simulink model "Simple_4Quad_payload_02"  (R2018b)
settings: Solver=VariableStepAuto  StartTime=0.0  StopTime=60  RelTol=1e-3
InitFcn:
  | Simple_4Quad_payload_02_const
values from neighbouring files (symbols this model uses):
  d1 = 0.25    [Colab_4Quad_model_01_const.m]    (also in Colab_4Quad_model_02_const.m = 0.5; Simple_4Quad_payload_01_const.m = 1; Simple_4Quad_payload_02_const.m = 1; Simple_4Quad_payload_03_const.m = 1)
  d2 = 0.25    [Colab_4Quad_model_01_const.m]    (also in Colab_4Quad_model_02_const.m = 0.5; Simple_4Quad_payload_01_const.m = 1; Simple_4Quad_payload_02_const.m = 1; Simple_4Quad_payload_03_const.m = 1)
  Des_rel_dist = 2    [Simple_4Quad_payload_01_const.m]    (also in Simple_4Quad_payload_02_const.m = 4; Simple_4Quad_payload_03_const.m = 4; Simple_4Quad_payload_04_const.m; Simple_4Quad_payload_05_const.m)
  g = 9.81    [Colab_4Quad_model_01_const.m]    (also in Colab_4Quad_model_02_const.m; Simple_2Quad_payload_01_const.m; Simple_2Quad_payload_02_const.m; Simple_2Quad_payload_03_const.m)
  Ix = 0.166667    [Colab_4Quad_model_01_const.m]    (also in Colab_4Quad_model_02_const.m = 0.02; Simple_4Quad_payload_01_const.m = 1; Simple_4Quad_payload_02_const.m = 1; Simple_4Quad_payload_03_const.m = 1)
  Iy = 0.166667    [Colab_4Quad_model_01_const.m]    (also in Colab_4Quad_model_02_const.m = 0.02; Simple_4Quad_payload_01_const.m = 1; Simple_4Quad_payload_02_const.m = 1; Simple_4Quad_payload_03_const.m = 1)
  Iz = 0.166667    [Colab_4Quad_model_01_const.m]    (also in Colab_4Quad_model_02_const.m = 0.02; Simple_4Quad_payload_01_const.m = 1; Simple_4Quad_payload_02_const.m = 1; Simple_4Quad_payload_03_const.m = 1)
  ki1_N = 0    [Simple_4Quad_payload_02_const.m]    (also in Simple_4Quad_payload_03_const.m; Simple_4Quad_payload_04_const.m; Simple_4Quad_payload_05_const.m; Simple_4Quad_payload_06_const.m)
  ki1_S = 0    [Simple_4Quad_payload_02_const.m]    (also in Simple_4Quad_payload_03_const.m; Simple_4Quad_payload_04_const.m)
  ki2_N = 0    [Simple_4Quad_payload_02_const.m]    (also in Simple_4Quad_payload_03_const.m; Simple_4Quad_payload_04_const.m; Simple_4Quad_payload_05_const.m; Simple_4Quad_payload_06_const.m = 10)
  ki2_S = 0    [Simple_4Quad_payload_02_const.m]    (also in Simple_4Quad_payload_03_const.m; Simple_4Quad_payload_04_const.m)
  kp1_N = 10    [Simple_4Quad_payload_02_const.m]    (also in Simple_4Quad_payload_03_const.m; Simple_4Quad_payload_04_const.m; Simple_4Quad_payload_05_const.m = 1; Simple_4Quad_payload_06_const.m = 1)
  kp1_S = 10    [Simple_4Quad_payload_02_const.m]    (also in Simple_4Quad_payload_03_const.m; Simple_4Quad_payload_04_const.m)
  kp2_N = 100    [Simple_4Quad_payload_02_const.m]    (also in Simple_4Quad_payload_03_const.m; Simple_4Quad_payload_04_const.m; Simple_4Quad_payload_05_const.m = 1; Simple_4Quad_payload_06_const.m = 1)
  kp2_S = 100    [Simple_4Quad_payload_02_const.m]    (also in Simple_4Quad_payload_03_const.m; Simple_4Quad_payload_04_const.m)
  l = 3.1819    [Colab_4Quad_model_01_const.m]    (also in Colab_4Quad_model_02_const.m = 3; Simple_2Quad_payload_04_const.m = 1; Simple_4Quad_payload_01_const.m = 1; Simple_4Quad_payload_02_const.m = 2)
  m = 1.5    [Colab_4Quad_model_01_const.m]    (also in Colab_4Quad_model_02_const.m; Simple_2Quad_payload_04_const.m = 1; Simple_4Quad_payload_01_const.m = 1; Simple_4Quad_payload_02_const.m = 1)
  M = 1.0    (= 1)    [Colab_4Quad_model_01_const.m]    (also in Colab_4Quad_model_02_const.m; Simple_2Quad_payload_01_const.m; Simple_2Quad_payload_02_const.m; Simple_2Quad_payload_03_const.m)
  Md = 1*[1;1;1]    [Simple_2Quad_payload_04_const.m]    (also in Simple_4Quad_payload_01_const.m = 1*[1;1;1;1;1;1]; Simple_4Quad_payload_02_const.m = 1*[1;1;1;1;1;1]; Simple_4Quad_payload_03_const.m = 1*[1;1;1;1;1;1]; Simple_4Quad_payload_04_const.m = 1*[1;1;1;1;1;1])
libraries: simulink x16
(part 2 of 2)

== system Simple_4Quad_payload_02/Agent4/PID_alpha4 ==
  alpha4_des : Inport
  alpha4 : Inport  Port=2
  D_alpha4 : Inport  Port=3
  PID Controller : simulink/Continuous/PID Controller  Controller=PID  Form=Parallel  TimeDomain=Continuous-time  SampleTime=-1  IntegratorMethod=Forward Euler  FilterMethod=Forward Euler  ControllerParametersSource=internal  P=kp1_N  I=ki1_N  D=0  UseFilter=on  N=100  TunerSelectOption=Transfer Function Based (PID Tuner App)  InitialConditionSource=internal  InitialConditionForIntegrator=0  InitialConditionForFilter=0  DifferentiatorICPrevScaledInput=0  ExternalReset=none  TrackingMode=off  Kt=1  LimitOutput=off  UpperSaturationLimit=inf  LowerSaturationLimit=-inf  LinearizeAsGain=on  AntiWindupMode=none  Kb=1  POutMin=[]  POutMax=[]  IOutMin=[]  IOutMax=[]  DOutMin=[]  DOutMax=[]  NOutMin=[]  NOutMax=[]  SumOutMin=[]  SumOutMax=[]  SaturationOutMin=[]  SaturationOutMax=[]  PParamMin=[]  PParamMax=[]  IParamMin=[]  IParamMax=[]  DParamMin=[]  DParamMax=[]  NParamMin=[]  NParamMax=[]  KbParamMin=[]  KbParamMax=[]  KtParamMin=[]  KtParamMax=[]  KbOutMin=[]  KbOutMax=[]  KtOutMin=[]  KtOutMax=[]  IntegratorOutMin=[]  IntegratorOutMax=[]  FilterOutMin=[]  FilterOutMax=[]  SumI1OutMin=[]  SumI1OutMax=[]  SumI2OutMin=[]  SumI2OutMax=[]  SumI3OutMin=[]  SumI3OutMax=[]  SumI4OutMin=[]  SumI4OutMax=[]  SumDOutMin=[]  SumDOutMax=[]  DifferentiatorOutMin=[]  DifferentiatorOutMax=[]  FilterDiffOutCoefMin=[]  FilterDiffOutCoefMax=[]  ReciprocalOutMin=[]  ReciprocalOutMax=[]  SumDenOutMin=[]  SumDenOutMax=[]  SumNumOutMin=[]  SumNumOutMax=[]  DivideOutMin=[]  DivideOutMax=[]  IntegratorContinuousStateAttributes=''  IntegratorStateMustResolveToSignalObject=off  IntegratorRTWStateStorageClass=Auto  FilterContinuousStateAttributes=''  FilterStateMustResolveToSignalObject=off  FilterRTWStateStorageClass=Auto  ParallelPVariant=InternalParameters  IdealPVariant=Disabled  IVariant=InternalParameters  DVariant=InternalParameters  IntegratorVariant=Continuous  SatVariant=Disabled  AWVariant=Passthrough  PCopyVariant=Disabled  TRVariant=Disabled  FdbkBlocksVariant=Forward  IdealPFdbkVariant=Disabled  SatFdbkVariant=Disabled  DerivativeFilterVariant=ContFilter  NVariant=InternalParameters  NCopyVariant=Disabled  FilterICVariant=InternalICsFilter  IntegratorICVariant=InternalICs  ExternalResetVariant=Disabled  TRSumVariant=Passthrough  SumFdbkVariant=Disabled  SumVariant=Sum_PID
  PID Controller1 : simulink/Continuous/PID Controller  Controller=PID  Form=Parallel  TimeDomain=Continuous-time  SampleTime=-1  IntegratorMethod=Forward Euler  FilterMethod=Forward Euler  ControllerParametersSource=internal  P=kp2_N  I=ki2_N  D=0  UseFilter=on  N=100  TunerSelectOption=Transfer Function Based (PID Tuner App)  InitialConditionSource=internal  InitialConditionForIntegrator=0  InitialConditionForFilter=0  DifferentiatorICPrevScaledInput=0  ExternalReset=none  TrackingMode=off  Kt=1  LimitOutput=off  UpperSaturationLimit=inf  LowerSaturationLimit=-inf  LinearizeAsGain=on  AntiWindupMode=none  Kb=1  POutMin=[]  POutMax=[]  IOutMin=[]  IOutMax=[]  DOutMin=[]  DOutMax=[]  NOutMin=[]  NOutMax=[]  SumOutMin=[]  SumOutMax=[]  SaturationOutMin=[]  SaturationOutMax=[]  PParamMin=[]  PParamMax=[]  IParamMin=[]  IParamMax=[]  DParamMin=[]  DParamMax=[]  NParamMin=[]  NParamMax=[]  KbParamMin=[]  KbParamMax=[]  KtParamMin=[]  KtParamMax=[]  KbOutMin=[]  KbOutMax=[]  KtOutMin=[]  KtOutMax=[]  IntegratorOutMin=[]  IntegratorOutMax=[]  FilterOutMin=[]  FilterOutMax=[]  SumI1OutMin=[]  SumI1OutMax=[]  SumI2OutMin=[]  SumI2OutMax=[]  SumI3OutMin=[]  SumI3OutMax=[]  SumI4OutMin=[]  SumI4OutMax=[]  SumDOutMin=[]  SumDOutMax=[]  DifferentiatorOutMin=[]  DifferentiatorOutMax=[]  FilterDiffOutCoefMin=[]  FilterDiffOutCoefMax=[]  ReciprocalOutMin=[]  ReciprocalOutMax=[]  SumDenOutMin=[]  SumDenOutMax=[]  SumNumOutMin=[]  SumNumOutMax=[]  DivideOutMin=[]  DivideOutMax=[]  IntegratorContinuousStateAttributes=''  IntegratorStateMustResolveToSignalObject=off  IntegratorRTWStateStorageClass=Auto  FilterContinuousStateAttributes=''  FilterStateMustResolveToSignalObject=off  FilterRTWStateStorageClass=Auto  ParallelPVariant=InternalParameters  IdealPVariant=Disabled  IVariant=InternalParameters  DVariant=InternalParameters  IntegratorVariant=Continuous  SatVariant=Disabled  AWVariant=Passthrough  PCopyVariant=Disabled  TRVariant=Disabled  FdbkBlocksVariant=Forward  IdealPFdbkVariant=Disabled  SatFdbkVariant=Disabled  DerivativeFilterVariant=ContFilter  NVariant=InternalParameters  NCopyVariant=Disabled  FilterICVariant=InternalICsFilter  IntegratorICVariant=InternalICs  ExternalResetVariant=Disabled  TRSumVariant=Passthrough  SumFdbkVariant=Disabled  SumVariant=Sum_PID
  Scope3 : Scope  NumInputPorts=3
  Sum : Sum  Inputs=|+-
  Sum1 : Sum  Inputs=|+-
  N4 : Outport
  wires:
  D_alpha4/1 -> Sum1/2
  alpha4/1 -> Sum/2
  alpha4_des/1 -> Sum/1
  Sum1/1 -> PID Controller1/1, Scope3/2
  Sum/1 -> PID Controller/1, Scope3/1
  PID Controller1/1 -> Scope3/3, N4/1
  PID Controller/1 -> Sum1/1

== system Simple_4Quad_payload_02/Agent4/PID_beta4 ==
  beta4_des : Inport
  beta4 : Inport  Port=2
  D_beta4 : Inport  Port=3
  PID Controller : simulink/Continuous/PID Controller  Controller=PID  Form=Parallel  TimeDomain=Continuous-time  SampleTime=-1  IntegratorMethod=Forward Euler  FilterMethod=Forward Euler  ControllerParametersSource=internal  P=kp1_S  I=ki1_S  D=0  UseFilter=on  N=100  TunerSelectOption=Transfer Function Based (PID Tuner App)  InitialConditionSource=internal  InitialConditionForIntegrator=0  InitialConditionForFilter=0  DifferentiatorICPrevScaledInput=0  ExternalReset=none  TrackingMode=off  Kt=1  LimitOutput=off  UpperSaturationLimit=inf  LowerSaturationLimit=-inf  LinearizeAsGain=on  AntiWindupMode=none  Kb=1  POutMin=[]  POutMax=[]  IOutMin=[]  IOutMax=[]  DOutMin=[]  DOutMax=[]  NOutMin=[]  NOutMax=[]  SumOutMin=[]  SumOutMax=[]  SaturationOutMin=[]  SaturationOutMax=[]  PParamMin=[]  PParamMax=[]  IParamMin=[]  IParamMax=[]  DParamMin=[]  DParamMax=[]  NParamMin=[]  NParamMax=[]  KbParamMin=[]  KbParamMax=[]  KtParamMin=[]  KtParamMax=[]  KbOutMin=[]  KbOutMax=[]  KtOutMin=[]  KtOutMax=[]  IntegratorOutMin=[]  IntegratorOutMax=[]  FilterOutMin=[]  FilterOutMax=[]  SumI1OutMin=[]  SumI1OutMax=[]  SumI2OutMin=[]  SumI2OutMax=[]  SumI3OutMin=[]  SumI3OutMax=[]  SumI4OutMin=[]  SumI4OutMax=[]  SumDOutMin=[]  SumDOutMax=[]  DifferentiatorOutMin=[]  DifferentiatorOutMax=[]  FilterDiffOutCoefMin=[]  FilterDiffOutCoefMax=[]  ReciprocalOutMin=[]  ReciprocalOutMax=[]  SumDenOutMin=[]  SumDenOutMax=[]  SumNumOutMin=[]  SumNumOutMax=[]  DivideOutMin=[]  DivideOutMax=[]  IntegratorContinuousStateAttributes=''  IntegratorStateMustResolveToSignalObject=off  IntegratorRTWStateStorageClass=Auto  FilterContinuousStateAttributes=''  FilterStateMustResolveToSignalObject=off  FilterRTWStateStorageClass=Auto  ParallelPVariant=InternalParameters  IdealPVariant=Disabled  IVariant=InternalParameters  DVariant=InternalParameters  IntegratorVariant=Continuous  SatVariant=Disabled  AWVariant=Passthrough  PCopyVariant=Disabled  TRVariant=Disabled  FdbkBlocksVariant=Forward  IdealPFdbkVariant=Disabled  SatFdbkVariant=Disabled  DerivativeFilterVariant=ContFilter  NVariant=InternalParameters  NCopyVariant=Disabled  FilterICVariant=InternalICsFilter  IntegratorICVariant=InternalICs  ExternalResetVariant=Disabled  TRSumVariant=Passthrough  SumFdbkVariant=Disabled  SumVariant=Sum_PID
  PID Controller1 : simulink/Continuous/PID Controller  Controller=PID  Form=Parallel  TimeDomain=Continuous-time  SampleTime=-1  IntegratorMethod=Forward Euler  FilterMethod=Forward Euler  ControllerParametersSource=internal  P=kp2_S  I=ki2_S  D=0  UseFilter=on  N=100  TunerSelectOption=Transfer Function Based (PID Tuner App)  InitialConditionSource=internal  InitialConditionForIntegrator=0  InitialConditionForFilter=0  DifferentiatorICPrevScaledInput=0  ExternalReset=none  TrackingMode=off  Kt=1  LimitOutput=off  UpperSaturationLimit=inf  LowerSaturationLimit=-inf  LinearizeAsGain=on  AntiWindupMode=none  Kb=1  POutMin=[]  POutMax=[]  IOutMin=[]  IOutMax=[]  DOutMin=[]  DOutMax=[]  NOutMin=[]  NOutMax=[]  SumOutMin=[]  SumOutMax=[]  SaturationOutMin=[]  SaturationOutMax=[]  PParamMin=[]  PParamMax=[]  IParamMin=[]  IParamMax=[]  DParamMin=[]  DParamMax=[]  NParamMin=[]  NParamMax=[]  KbParamMin=[]  KbParamMax=[]  KtParamMin=[]  KtParamMax=[]  KbOutMin=[]  KbOutMax=[]  KtOutMin=[]  KtOutMax=[]  IntegratorOutMin=[]  IntegratorOutMax=[]  FilterOutMin=[]  FilterOutMax=[]  SumI1OutMin=[]  SumI1OutMax=[]  SumI2OutMin=[]  SumI2OutMax=[]  SumI3OutMin=[]  SumI3OutMax=[]  SumI4OutMin=[]  SumI4OutMax=[]  SumDOutMin=[]  SumDOutMax=[]  DifferentiatorOutMin=[]  DifferentiatorOutMax=[]  FilterDiffOutCoefMin=[]  FilterDiffOutCoefMax=[]  ReciprocalOutMin=[]  ReciprocalOutMax=[]  SumDenOutMin=[]  SumDenOutMax=[]  SumNumOutMin=[]  SumNumOutMax=[]  DivideOutMin=[]  DivideOutMax=[]  IntegratorContinuousStateAttributes=''  IntegratorStateMustResolveToSignalObject=off  IntegratorRTWStateStorageClass=Auto  FilterContinuousStateAttributes=''  FilterStateMustResolveToSignalObject=off  FilterRTWStateStorageClass=Auto  ParallelPVariant=InternalParameters  IdealPVariant=Disabled  IVariant=InternalParameters  DVariant=InternalParameters  IntegratorVariant=Continuous  SatVariant=Disabled  AWVariant=Passthrough  PCopyVariant=Disabled  TRVariant=Disabled  FdbkBlocksVariant=Forward  IdealPFdbkVariant=Disabled  SatFdbkVariant=Disabled  DerivativeFilterVariant=ContFilter  NVariant=InternalParameters  NCopyVariant=Disabled  FilterICVariant=InternalICsFilter  IntegratorICVariant=InternalICs  ExternalResetVariant=Disabled  TRSumVariant=Passthrough  SumFdbkVariant=Disabled  SumVariant=Sum_PID
  Scope3 : Scope  NumInputPorts=3
  Sum : Sum  Inputs=|+-
  Sum1 : Sum  Inputs=|+-
  S4 : Outport
  wires:
  D_beta4/1 -> Sum1/2
  PID Controller/1 -> Sum1/1
  PID Controller1/1 -> S4/1, Scope3/3
  Sum/1 -> PID Controller/1, Scope3/1
  Sum1/1 -> PID Controller1/1, Scope3/2
  beta4_des/1 -> Sum/1
  beta4/1 -> Sum/2

== matlab function Simple_4Quad_payload_02/payload/Controller ==
  data: e input; F output; Alpha_Des output; PHI input; Beta_Des output; Md parameter; g parameter; M parameter; OUT output; d1 parameter; d2 parameter; Ix parameter; Iy parameter; Iz parameter; l parameter; Des_rel_dist parameter; B output; U output
function [F,Alpha_Des,Beta_Des,OUT,B,U] = fcn(e,PHI, Md, g, M, d1, d2, Ix, Iy, Iz, l, Des_rel_dist)

phi = PHI(1);
theta = PHI(2);
psi = PHI(3);

Io = diag([Ix;Iy;Iz]);

Ro = [cos(psi)*cos(theta) cos(psi)*sin(theta)*sin(phi)-sin(psi)*cos(phi) cos(psi)*sin(theta)*cos(phi)+sin(psi)*sin(phi);
    sin(psi)*cos(theta) sin(psi)*sin(theta)*sin(phi)+cos(psi)*cos(phi) sin(psi)*sin(theta)*cos(phi)-cos(psi)*sin(phi);
    -sin(theta) cos(theta)*sin(phi) cos(theta)*cos(phi)];

s1 = [0 0 0;
    0 0 -d1;
    0 d1 0];

s2 = [0 0 0;
    0 0 d1;
    0 -d1 0];

s3 = [0 0 d2;
    0 0 0;
    -d2 0 0];

s4 = [0 0 -d2;
    0 0 0;
    d2 0 0];

B = [(1/M)*Ro (1/M)*Ro (1/M)*Ro (1/M)*Ro;
    Io^(-1)*s1 Io^(-1)*s2 Io^(-1)*s3 Io^(-1)*s4;
    1 0 0 1 0 0 0 0 0 0 0 0;
    0 0 0 0 0 0 0 1 0 0 1 0;
    1 0 0 0 0 0 0 0 0 0 0 0;
    0 0 0 0 0 0 0 1 0 0 0 0];

D = [0;0;-g;0;0;0];

SGN = zeros(6);
for i=1:6
    SGN(i,i) = e(i)/(abs(e(i))+0.1);
end

Z = SGN*Md;
U = Z - D;

u_t = U(1:3);
rx_des = Des_rel_dist;
ry_des = Des_rel_dist;
q1 = (rx_des - (2*d1)) / (2*l);
q2 = (ry_des - (2*d2)) / (2*l);
K1 = sqrt( ((u_t(2)/2)^2 + (u_t(3)/4)^2) / ((1/(q1^2))-1) );
K2 = sqrt( ((u_t(1)/2)^2 + (u_t(3)/4)^2) / ((1/(q2^2))-1) );

U_gen = [U;0;0;K1;K2];

Mu = B' * (B*B')^(-1) * U_gen;

F = zeros(4,1);
Alpha_Des = zeros(4,1);
Beta_Des = zeros(4,1);

for i=1:4
    F(i,1) = sqrt( Mu((3*(i-1)+1):(3*(i-1)+3))'*Mu((3*(i-1)+1):(3*(i-1)+3)) );
    Alpha_Des(i,1) = asin( Mu(3*(i-1)+3,1)/F(i,1) );
    Beta_Des(i,1) = atan2( Mu(3*(i-1)+2,1),Mu(3*(i-1)+1,1) );
    if Beta_Des(i,1) < (-3*pi/4)
        Beta_Des(i,1) = 2*pi + Beta_Des(i,1);
    end
end

OUT = U;

end

== matlab function Simple_4Quad_payload_02/payload/Dynamic Model ==
  data: fs input; DD_PHI output; D_PHI output; D_omega_o output; alphas input; betas input; PHI input; omega_o input; DD_P output; d2 parameter; M parameter; Ix parameter; g parameter; Iy parameter; Iz parameter; d1 parameter; R1 output; R2 output; R3 output; R4 output; Ro output
function [DD_PHI,D_PHI,D_omega_o,DD_P,R1,R2,R3,R4,Ro] = fcn(fs,alphas,betas,PHI,omega_o,d2, M, Ix,g, Iy, Iz, d1)

f1 = fs(1);
f2 = fs(2);
f3 = fs(3);
f4 = fs(4);

alpha1 = alphas(1);
alpha2 = alphas(2);
alpha3 = alphas(3);
alpha4 = alphas(4);

beta1 = betas(1);
beta2 = betas(2);
beta3 = betas(3);
beta4 = betas(4);

phi = PHI(1);
theta = PHI(2);
psi = PHI(3);

Io = diag([Ix;Iy;Iz]);

R1 = [cos(alpha1)*cos(beta1) -sin(beta1) -sin(alpha1)*cos(beta1);
    cos(alpha1)*sin(beta1) cos(beta1) -sin(alpha1)*sin(beta1);
    sin(alpha1) 0 cos(alpha1)];

R2 = [cos(alpha2)*cos(beta2) -sin(beta2) -sin(alpha2)*cos(beta2);
    cos(alpha2)*sin(beta2) cos(beta2) -sin(alpha2)*sin(beta2);
    sin(alpha2) 0 cos(alpha2)];

R3 = [cos(alpha3)*cos(beta3) -sin(beta3) -sin(alpha3)*cos(beta3);
    cos(alpha3)*sin(beta3) cos(beta3) -sin(alpha3)*sin(beta3);
    sin(alpha3) 0 cos(alpha3)];

R4 = [cos(alpha4)*cos(beta4) -sin(beta4) -sin(alpha4)*cos(beta4);
    cos(alpha4)*sin(beta4) cos(beta4) -sin(alpha4)*sin(beta4);
    sin(alpha4) 0 cos(alpha4)];

Ro = [cos(psi)*cos(theta) cos(psi)*sin(theta)*sin(phi)-sin(psi)*cos(phi) cos(psi)*sin(theta)*cos(phi)+sin(psi)*sin(phi);
    sin(psi)*cos(theta) sin(psi)*sin(theta)*sin(phi)+cos(psi)*cos(phi) sin(psi)*sin(theta)*cos(phi)-cos(psi)*sin(phi);
    -sin(theta) cos(theta)*sin(phi) cos(theta)*cos(phi)];

F1 = [f1;0;0];
F2 = [f2;0;0];
F3 = [f3;0;0];
F4 = [f4;0;0];

r1 = [d1;0;0];
r2 = [-d1;0;0];
r3 = [0;d2;0];
r4 = [0;-d2;0];

G = [0;0;-g];

D_omega_o = (Io^(-1)) * ( ( External_Product3(r1,F1) + External_Product3(r2,F2) + External_Product3(r3,F3) + External_Product3(r4,F4) ) - External_Product3(omega_o,(Io*omega_o)) );
DD_P = (1/M) * ( ( Ro * ( R1*F1 + R2*F2 + R3*F3 + R4*F4 ) ) + M*G );

R_phi_o = [1 0 -sin(theta);
    0 cos(phi) cos(theta)*sin(phi);
    0 -sin(phi) cos(theta)*cos(phi)];

D_PHI = (R_phi_o^-1) * omega_o;

DR_phi_o = [0 0 -D_PHI(2)*cos(theta);
    0 -D_PHI(1)*sin(phi) (-D_PHI(2)*sin(theta)*sin(phi))+(D_PHI(1)*cos(theta)*cos(phi));
    0 -D_PHI(1)*cos(phi) (-D_PHI(2)*sin(theta)*cos(phi))-(D_PHI(1)*cos(theta)*sin(phi))];

DD_PHI = DR_phi_o * omega_o + R_phi_o * D_omega_o;

end

== matlab function Simple_4Quad_payload_02/Agent2/Dynamic Model2 ==
  data: DD_alpha2 output; N2 input; S2 input; f2 input; alpha2 input; beta2 input; D_alpha2 input; D_beta2 input; m parameter; g parameter; DD_PHI input; DD_P input; D_PHI input; l parameter; d1 parameter; PHI input; DD_beta2 output; U2 output; Po input; P2 output
function [DD_alpha2,DD_beta2,U2,P2]  = fcn(N2,S2,f2,alpha2,beta2,D_alpha2,D_beta2,m, g,DD_PHI,DD_P,D_PHI, l, d1,PHI,Po)

phi = PHI(1);
theta = PHI(2);
psi = PHI(3);

Dist2_local = [-d1;0;0];
D2_angles = [0;D_alpha2;D_beta2];

Ro = [cos(psi)*cos(theta) cos(psi)*sin(theta)*sin(phi)-sin(psi)*cos(phi) cos(psi)*sin(theta)*cos(phi)+sin(psi)*sin(phi);
    sin(psi)*cos(theta) sin(psi)*sin(theta)*sin(phi)+cos(psi)*cos(phi) sin(psi)*sin(theta)*cos(phi)-cos(psi)*sin(phi);
    -sin(theta) cos(theta)*sin(phi) cos(theta)*cos(phi)];

R2 = [cos(alpha2)*cos(beta2) -sin(beta2) -sin(alpha2)*cos(beta2);
    cos(alpha2)*sin(beta2) cos(beta2) -sin(alpha2)*sin(beta2);
    sin(alpha2) 0 cos(alpha2)];

C1_2 = External_Product3(D_PHI,Dist2_local);
C2_2 = External_Product3(D_PHI,C1_2);
C3_2 = External_Product3(DD_PHI,Dist2_local);

C4_2 = External_Product3(D2_angles,Dist2_local);
C5_2 = External_Product3(D2_angles,C4_2);

a2_part = (  R2' * ( Ro'*DD_P + C2_2 + C3_2 ) ) + C5_2;

G2_local = R2' * Ro' * [0;0;-g];

T2 = m*a2_part(1) + f2 - m*G2_local(1);
DD_alpha2 = (1/m/l) * (N2 - m*a2_part(2) + m*G2_local(2));
DD_beta2 = (1/m/l) * (S2 - m*a2_part(3) + m*G2_local(3));

U2 = Ro * R2 * [T2;S2;N2];

P2 = Po + Ro*Dist2_local + Ro*R2*[l;0;0];

end

== matlab function Simple_4Quad_payload_02/Agent1 /Dynamic Model1 ==
  data: DD_alpha1 output; N1 input; S1 input; f1 input; alpha1 input; beta1 input; D_alpha1 input; D_beta1 input; m parameter; g parameter; DD_PHI input; DD_P input; D_PHI input; l parameter; d1 parameter; PHI input; DD_beta1 output; U1 output; Po input; P1 output
function [DD_alpha1,DD_beta1,U1,P1]  = fcn(N1,S1,f1,alpha1,beta1,D_alpha1,D_beta1,m, g,DD_PHI,DD_P,D_PHI, l, d1,PHI,Po)

phi = PHI(1);
theta = PHI(2);
psi = PHI(3);

Dist1_local = [d1;0;0];
D1_angles = [0;D_alpha1;D_beta1];

Ro = [cos(psi)*cos(theta) cos(psi)*sin(theta)*sin(phi)-sin(psi)*cos(phi) cos(psi)*sin(theta)*cos(phi)+sin(psi)*sin(phi);
    sin(psi)*cos(theta) sin(psi)*sin(theta)*sin(phi)+cos(psi)*cos(phi) sin(psi)*sin(theta)*cos(phi)-cos(psi)*sin(phi);
    -sin(theta) cos(theta)*sin(phi) cos(theta)*cos(phi)];

R1 = [cos(alpha1)*cos(beta1) -sin(beta1) -sin(alpha1)*cos(beta1);
    cos(alpha1)*sin(beta1) cos(beta1) -sin(alpha1)*sin(beta1);
    sin(alpha1) 0 cos(alpha1)];

C1_1 = External_Product3(D_PHI,Dist1_local);
C2_1 = External_Product3(D_PHI,C1_1);
C3_1 = External_Product3(DD_PHI,Dist1_local);

C4_1 = External_Product3(D1_angles,Dist1_local);
C5_1 = External_Product3(D1_angles,C4_1);

a1_part = (  R1' * ( Ro'*DD_P + C2_1 + C3_1 ) ) + C5_1;

G1_local = R1' * Ro' * [0;0;-g];

T1 = m*a1_part(1) + f1 - m*G1_local(1);
DD_alpha1 = (1/m/l) * (N1 - m*a1_part(2) + m*G1_local(2));
DD_beta1 = (1/m/l) * (S1 - m*a1_part(3) + m*G1_local(3));

U1 = Ro * R1 * [T1;S1;N1];

P1 = Po + Ro*Dist1_local + Ro*R1*[l;0;0];

end

== matlab function Simple_4Quad_payload_02/Agent4/Dynamic Model4 ==
  data: DD_alpha4 output; N4 input; S4 input; f4 input; alpha4 input; beta4 input; D_alpha4 input; D_beta4 input; m parameter; g parameter; DD_PHI input; DD_P input; D_PHI input; l parameter; d2 parameter; PHI input; DD_beta4 output; U4 output; Po input; P4 output
function [DD_alpha4,DD_beta4,U4,P4]  = fcn(N4,S4,f4,alpha4,beta4,D_alpha4,D_beta4,m, g,DD_PHI,DD_P,D_PHI, l, d2,PHI,Po)

phi = PHI(1);
theta = PHI(2);
psi = PHI(3);

Dist4_local = [0;-d2;0];
D4_angles = [0;D_alpha4;D_beta4];

Ro = [cos(psi)*cos(theta) cos(psi)*sin(theta)*sin(phi)-sin(psi)*cos(phi) cos(psi)*sin(theta)*cos(phi)+sin(psi)*sin(phi);
    sin(psi)*cos(theta) sin(psi)*sin(theta)*sin(phi)+cos(psi)*cos(phi) sin(psi)*sin(theta)*cos(phi)-cos(psi)*sin(phi);
    -sin(theta) cos(theta)*sin(phi) cos(theta)*cos(phi)];

R4 = [cos(alpha4)*cos(beta4) -sin(beta4) -sin(alpha4)*cos(beta4);
    cos(alpha4)*sin(beta4) cos(beta4) -sin(alpha4)*sin(beta4);
    sin(alpha4) 0 cos(alpha4)];

C1_4 = External_Product3(D_PHI,Dist4_local);
C2_4 = External_Product3(D_PHI,C1_4);
C3_4 = External_Product3(DD_PHI,Dist4_local);

C4_4 = External_Product3(D4_angles,Dist4_local);
C5_4 = External_Product3(D4_angles,C4_4);

a4_part = (  R4' * ( Ro'*DD_P + C2_4 + C3_4 ) ) + C5_4;

G4_local = R4' * Ro' * [0;0;-g];

T4 = m*a4_part(1) + f4 - m*G4_local(1);
DD_alpha4 = (1/m/l) * (N4 - m*a4_part(2) + m*G4_local(2));
DD_beta4 = (1/m/l) * (S4 - m*a4_part(3) + m*G4_local(3));

U4 = Ro * R4 * [T4;S4;N4];

P4 = Po + Ro*Dist4_local + Ro*R4*[l;0;0];

end

== matlab function Simple_4Quad_payload_02/Agent3/Dynamic Model3 ==
  data: DD_alpha3 output; N3 input; S3 input; f3 input; alpha3 input; beta3 input; D_alpha3 input; D_beta3 input; m parameter; g parameter; DD_PHI input; DD_P input; D_PHI input; l parameter; d2 parameter; PHI input; DD_beta3 output; U3 output; Po input; P3 output
function [DD_alpha3,DD_beta3,U3,P3]  = fcn(N3,S3,f3,alpha3,beta3,D_alpha3,D_beta3,m, g,DD_PHI,DD_P,D_PHI, l, d2,PHI,Po)

phi = PHI(1);
theta = PHI(2);
psi = PHI(3);

Dist3_local = [0;d2;0];
D3_angles = [0;D_alpha3;D_beta3];

Ro = [cos(psi)*cos(theta) cos(psi)*sin(theta)*sin(phi)-sin(psi)*cos(phi) cos(psi)*sin(theta)*cos(phi)+sin(psi)*sin(phi);
    sin(psi)*cos(theta) sin(psi)*sin(theta)*sin(phi)+cos(psi)*cos(phi) sin(psi)*sin(theta)*cos(phi)-cos(psi)*sin(phi);
    -sin(theta) cos(theta)*sin(phi) cos(theta)*cos(phi)];

R3 = [cos(alpha3)*cos(beta3) -sin(beta3) -sin(alpha3)*cos(beta3);
    cos(alpha3)*sin(beta3) cos(beta3) -sin(alpha3)*sin(beta3);
    sin(alpha3) 0 cos(alpha3)];

C1_3 = External_Product3(D_PHI,Dist3_local);
C2_3 = External_Product3(D_PHI,C1_3);
C3_3 = External_Product3(DD_PHI,Dist3_local);

C4_3 = External_Product3(D3_angles,Dist3_local);
C5_3 = External_Product3(D3_angles,C4_3);

a3_part = (  R3' * ( Ro'*DD_P + C2_3 + C3_3 ) ) + C5_3;

G3_local = R3' * Ro' * [0;0;-g];

T3 = m*a3_part(1) + f3 - m*G3_local(1);
DD_alpha3 = (1/m/l) * (N3 - m*a3_part(2) + m*G3_local(2));
DD_beta3 = (1/m/l) * (S3 - m*a3_part(3) + m*G3_local(3));

U3 = Ro * R3 * [T3;S3;N3];

P3 = Po + Ro*Dist3_local + Ro*R3*[l;0;0];

end

== matlab function Simple_4Quad_payload_02/Relative Positions observation/MATLAB Function ==
  data: P1 input; e_cons_1 output; P2 input; P3 input; P4 input; e_cons_2 output; e_cons_3 output; e_cons_4 output; Des_rel_dist parameter
function [e_cons_1,e_cons_2,e_cons_3,e_cons_4] = fcn(P1,P2,P3,P4,Des_rel_dist)

Pos_local_1 = [Des_rel_dist/2;0;0];
Pos_local_2 = [-Des_rel_dist/2;0;0];
Pos_local_3 = [0;Des_rel_dist/2;0];
Pos_local_4 = [0;-Des_rel_dist/2;0];

Pos_All = [P1 P2 P3 P4];
Pos_local_All = [Pos_local_1 Pos_local_2 Pos_local_3 Pos_local_4];
e_cons_All = zeros(3,4);

for i=1:4
    for j=1:4
        e_cons_All(:,i) = e_cons_All(:,i) + ( (Pos_All(:,i)-Pos_All(:,j)) - (Pos_local_All(:,i)-Pos_local_All(:,j)) );
    end
end

e_cons_1 = e_cons_All(:,1);
e_cons_2 = e_cons_All(:,2);
e_cons_3 = e_cons_All(:,3);
e_cons_4 = e_cons_All(:,4);

end

== matlab function Simple_4Quad_payload_02/payload/MATLAB Function ==
  data: t input; Vd output
function Vd = fcn(t)

fv = 0.2;
rv = 1;
Vdz = 0.2;
Vd = [rv*fv*sin(fv*t);
    -rv*fv*cos(fv*t);
    Vdz];

end
